simulink model "sled_syst_diskr"  (R2021b)
settings: Solver=VariableStepAuto  StartTime=0.0  StopTime=0.05  RelTol=1e-3
libraries: cstblocks x4
settings Model: Creator=Admin  LastModifiedBy=Admin

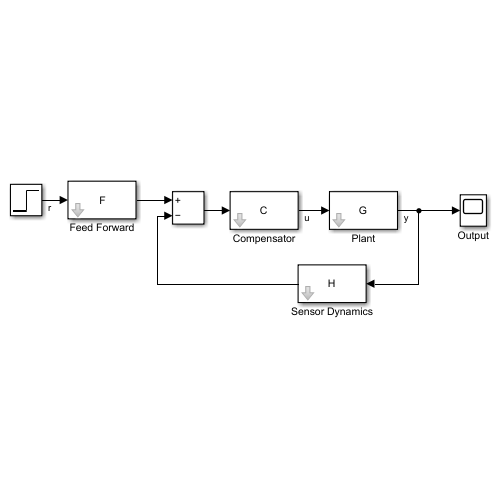
[thumbnail: Simulink's stored preview of the top-level diagram]
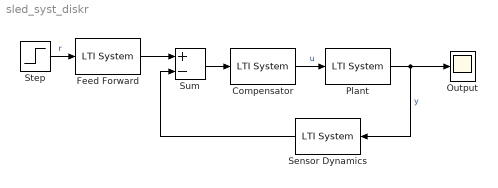
== system sled_syst_diskr ==
  Compensator : cstblocks/LTI System  sys=C  IC=[]
  Feed Forward : cstblocks/LTI System  sys=F  IC=[]
  Output : Scope
  Plant : cstblocks/LTI System  sys=G  IC=[]
  Sensor Dynamics : cstblocks/LTI System  sys=H  IC=[]
  Step : Step  Time=0  SampleTime=0
  Sum : Sum  Inputs=+-
  wires:
  Step/1 -> Feed Forward/1  "r"
  Feed Forward/1 -> Sum/1
  Sensor Dynamics/1 -> Sum/2
  Sum/1 -> Compensator/1
  Compensator/1 -> Plant/1  "u"
  Plant/1 -> Output/1, Sensor Dynamics/1  "y"
